simulink model "HESS"  (R2023a)
settings: Solver=daessc  StartTime=0.0  StopTime=1800  MaxStep=0.1  RelTol=1e-3
values from neighbouring files (symbols this model uses):
  Max_Power = 100000    [setHESSParam.m]    (also in setHESSParamv2.m)
  sim_case = i    [create_SOC_dataset.m]    (also in create_csv.m = 2; setHESSParam.m = 6; setHESSParamv2.m = 6)
undefined symbols (not defined in the file or in its folder): Battery, Capacitor, Ri
libraries: fl_lib x41, nesl_utility x22, rllib x2, dspstat3 x2, batteryecm_lib x1, autolibshared x1
(part 1 of 2)
settings Model: Creator=antaeug  LastModifiedBy=antaeug

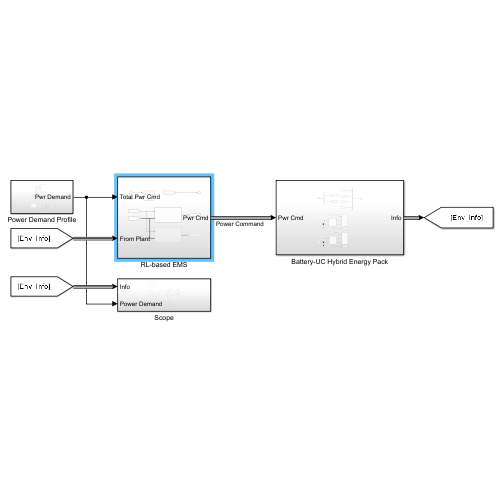
[thumbnail: Simulink's stored preview of the top-level diagram]
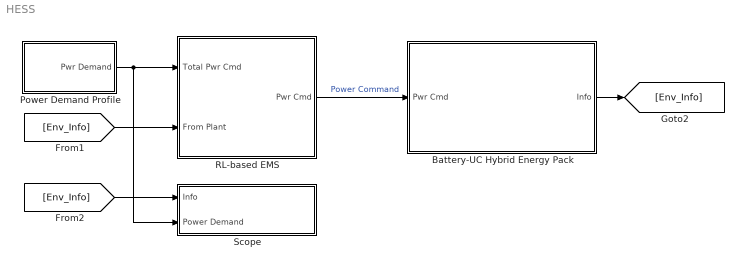
== system HESS ==
  Battery-UC Hybrid Energy Pack : Subsystem
  Power Demand Profile : Subsystem
  RL-based EMS : Subsystem
  Scope : Subsystem
  wires:
  Power Demand Profile/1(Pwr Demand) -> RL-based EMS/1(Total Pwr Cmd), Scope/2(Power Demand)
  RL-based EMS/1(Pwr Cmd) -> Battery-UC Hybrid Energy Pack/1(Pwr Cmd)  "Power Command"
  Battery-UC Hybrid Energy Pack/1(Info) -> [Env_Info]
  [Env_Info] -> Scope/1(Info)
  [Env_Info] -> RL-based EMS/2(From Plant)

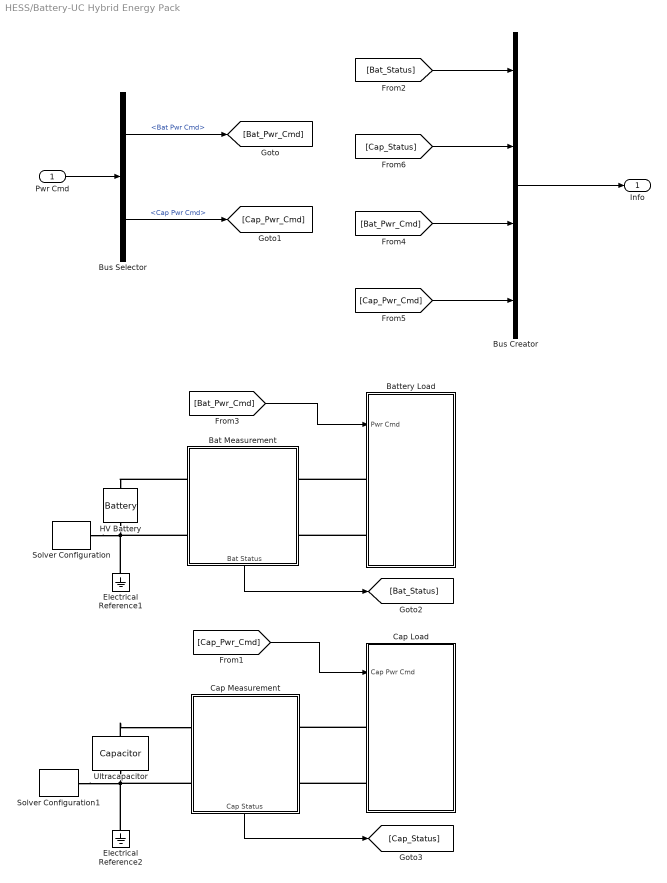
== system HESS/Battery-UC Hybrid Energy Pack ==
  Pwr Cmd : Inport
  Bat Measurement : Subsystem
      settings: PortSchema="{\"entries\":[{\"content\":{\"sides\":[{\"content\":{\"connectorIds\":[\"LConn1\",\"LConn2\"]},\"type\":\"ConnectorPlacement.EquallySpacedRectSide\",\"uuid\":\"d922d1f1-019d-451f-8be4-16b01e818775\"},{\"content\":{\"connectorIds\":[\"RConn1\",\"RConn2\"],\"side\":\"RIGHT\"},\"type\":\"ConnectorPlacement.EquallySpacedRectSide\",\"uuid\":\"6462d40f-4676-4bff-8e25-5b847feb4e24\"},{\"content\":{\"side\":\"TOP\"},\"type\":\"ConnectorPlacement.EquallySpacedRectSide\",\"uuid\":\"03ad4d94-013a-4b50-b094-3d1359848380\"},{\"content\":{\"connectorIds\":[\"Out1\"],\"side\":\"BOTTOM\"},\"type\":\"ConnectorPlacement.EquallySpacedRectSide\",\"uuid\":\"1e4082bc-bf86-4ee6-a4f5-78f09401198d\"}]},\"type\":\"ConnectorPlacement.EquallySpacedConnector\",\"uuid\":\"2964760f-0df3-43f8-9aa6-d9b794f3ad37\"}],\"packageUris\":[\"http://schema.mathworks.com/mf0/Connector/R2020b\"],\"version\":\"1.0\"}"
  Battery Load : Subsystem
  Bus Creator : BusCreator  Inputs=4
  Bus Selector : BusSelector  OutputSignals=Bat Pwr Cmd,Cap Pwr Cmd
  Cap Load : Subsystem
  Cap Measurement : Subsystem
      settings: PortSchema="{\"entries\":[{\"content\":{\"sides\":[{\"content\":{\"connectorIds\":[\"LConn1\",\"LConn2\"]},\"type\":\"ConnectorPlacement.EquallySpacedRectSide\",\"uuid\":\"d922d1f1-019d-451f-8be4-16b01e818775\"},{\"content\":{\"connectorIds\":[\"RConn1\",\"RConn2\"],\"side\":\"RIGHT\"},\"type\":\"ConnectorPlacement.EquallySpacedRectSide\",\"uuid\":\"6462d40f-4676-4bff-8e25-5b847feb4e24\"},{\"content\":{\"side\":\"TOP\"},\"type\":\"ConnectorPlacement.EquallySpacedRectSide\",\"uuid\":\"03ad4d94-013a-4b50-b094-3d1359848380\"},{\"content\":{\"connectorIds\":[\"Out1\"],\"side\":\"BOTTOM\"},\"type\":\"ConnectorPlacement.EquallySpacedRectSide\",\"uuid\":\"1e4082bc-bf86-4ee6-a4f5-78f09401198d\"}]},\"type\":\"ConnectorPlacement.EquallySpacedConnector\",\"uuid\":\"2964760f-0df3-43f8-9aa6-d9b794f3ad37\"}],\"packageUris\":[\"http://schema.mathworks.com/mf0/Connector/R2020b\"],\"version\":\"1.0\"}"
  Electrical Reference1 : fl_lib/Electrical/Electrical Elements/Electrical Reference
  Electrical Reference2 : fl_lib/Electrical/Electrical Elements/Electrical Reference
  HV Battery : batteryecm_lib/Battery  Vnom=Battery.NominalVoltage V  prm_dir=1  R1_dis=2 Ohm  R1_ch=2 Ohm  R1=Battery.InternalResistance Ohm  prm_AH=2  AH=Battery.Capacity hr*A  V1=Battery.V1 V  AH1=Battery.AH1 hr*A  prm_R2=simscape.enum.battery.prm_R2.disabled  R2=2000 Ohm  Tmeas=25 degC  charge_measurement_port=simscape.enum.battery.enable.no  prm_dyn=simscape.enum.battery.prm_dyn.off  Rp1=0.005 Ohm  tau1=30 s  Rp2=0.005 Ohm  tau2=30 s  Rp3=0.005 Ohm  tau3=30 s  Rp4=0.005 Ohm  tau4=30 s  Rp5=0.005 Ohm  tau5=30 s  prm_fade=simscape.enum.battery.prm_fade.disabled  N_fade=100  AH_fade=45 hr*A  R1_fade=2.02 Ohm  R1_ch_fade=2.02 Ohm  V1_fade=10.35 V  prm_age=simscape.enum.battery.prm_age.disabled  prm_age_OCV=1  OCV_age=0.9  SOC_age=60  Tmeas_age=298.15 K  delta_time_age_vec=[0] d  temperature_age_vec=[273] K  OCV_scaling_age=2.2134e6  OCV_offset_age=1.632e6  temp_exp_age=0.515833569 V  t_exp_age=0.75  Vnom_T2=Vnom V  R1_T2=Ri+0.1*Ri Ohm  R1_T2_dis=2.2 Ohm  R1_T2_ch=2.2 Ohm  V1_T2=V1 V  R2_T2=2200 Ohm  Rp1_T2=0.005 Ohm  tau1_T2=30 s  Rp2_T2=0.005 Ohm  tau2_T2=30 s  Rp3_T2=0.005 Ohm  tau3_T2=30 s  Rp4_T2=0.005 Ohm  tau4_T2=30 s  Rp5_T2=0.005 Ohm  tau5_T2=30 s  Tmeas2=0 degC  thermal_port=simscape.enum.thermaleffects.omit  thermal_mass=89400 J/K  i_specify=off  i_priority=None  i=0 A  i_nominal_specify=off  i_nominal_unit=A  i_nominal_value=1  v_specify=off  v_priority=None  v=0 V  v_nominal_specify=off  v_nominal_unit=V  v_nominal_value=1  charge_specify=on  charge_priority=High  charge=Battery.InitialCharge hr*A  charge_nominal_specify=off  charge_nominal_unit=A*hr  charge_nominal_value=1  num_cycles_specify=off  num_cycles_priority=High  num_cycles=0  num_cycles_nominal_specify=off  num_cycles_nominal_unit=1  num_cycles_nominal_value=1  temperature_specify=on  temperature_priority=High  temperature=25 degC  temperature_nominal_specify=off  temperature_nominal_unit=K  temperature_nominal_value=1
  Solver Configuration : nesl_utility/Solver Configuration  PhysicalDomain=network_engine_domain  SubClassName=solver  LeftPortType=input  RightPortType=generic  Tones=[]  Harmonics=[]  SimulateNoise=off  Profile=off  UseLocalSampling=off  EnableSwitchedLinearOptims=on  FrequencyDomain=off  UseCCode=off  RelTol=0.001  AbsTol=1e-06  MinStep=1e-09  ToWorkspace=off  RevertToSquareIcSolve=off  NumHomotopyIterations=100  PhasorMode=off  PhasorModeNumHarmonics=1  ConsistencySolver=NEWTON_FTOL  IndexReductionMethod=DerivativeReplacement  DoDC=off  ResidualTolerance=1e-09  ConsistencyTolSource=GLOBAL  ConsistencyAbsTol=0.001  ConsistencyRelTol=0.001  ConsistencyTolFactor=0.001  UseLocalSolver=on  LocalSolverChoice=NE_BACKWARD_EULER_ADVANCER  ResolveIndetEquations=on  FunctionEvalNumThread=1  LocalSolverSampleTime=0.01  DoFixedCost=on  MaxNonlinIter=3  MaxModeIter=2  ComputeImpulses=off  ImpulseIterations=2  LinearAlgebra=auto  LinearAlgebraNumThread=0  EquationFormulation=NE_TIME_EF  DelaysMemoryBudget=1024  AutomaticFiltering=on  FilteringTimeConstant=0.001  PartitionStorageMethod=AS_NEEDED  PartitionMemoryBudget=1024  PartitionMethod=FAST
  Solver Configuration1 : nesl_utility/Solver Configuration  PhysicalDomain=network_engine_domain  SubClassName=solver  LeftPortType=input  RightPortType=generic  Tones=[]  Harmonics=[]  SimulateNoise=off  Profile=off  UseLocalSampling=off  EnableSwitchedLinearOptims=on  FrequencyDomain=off  UseCCode=off  RelTol=0.001  AbsTol=1e-06  MinStep=1e-09  ToWorkspace=off  RevertToSquareIcSolve=off  NumHomotopyIterations=100  PhasorMode=off  PhasorModeNumHarmonics=1  ConsistencySolver=NEWTON_FTOL  IndexReductionMethod=DerivativeReplacement  DoDC=off  ResidualTolerance=1e-09  ConsistencyTolSource=GLOBAL  ConsistencyAbsTol=0.001  ConsistencyRelTol=0.001  ConsistencyTolFactor=0.001  UseLocalSolver=on  LocalSolverChoice=NE_BACKWARD_EULER_ADVANCER  ResolveIndetEquations=on  FunctionEvalNumThread=1  LocalSolverSampleTime=0.01  DoFixedCost=on  MaxNonlinIter=3  MaxModeIter=2  ComputeImpulses=off  ImpulseIterations=2  LinearAlgebra=auto  LinearAlgebraNumThread=0  EquationFormulation=NE_TIME_EF  DelaysMemoryBudget=1024  AutomaticFiltering=on  FilteringTimeConstant=0.001  PartitionStorageMethod=AS_NEEDED  PartitionMemoryBudget=1024  PartitionMethod=FAST
  Ultracapacitor : fl_lib/Electrical/Electrical Elements/Capacitor  c=Capacitor.Capacitance F  r=Capacitor.InternalResistance mOhm  g=0 1/Ohm  i_specify=off  i_priority=None  i=20 A  i_nominal_specify=off  i_nominal_unit=A  i_nominal_value=1  v_specify=off  v_priority=None  v=600 V  v_nominal_specify=off  v_nominal_unit=V  v_nominal_value=1  vc_specify=on  vc_priority=None  vc=Capacitor.Voltage V  vc_nominal_specify=off  vc_nominal_unit=V  vc_nominal_value=600
  Info : Outport
  wires:
  Pwr Cmd/1 -> Bus Selector/1
  Bus Selector/1 -> [Bat_Pwr_Cmd]  "<Bat Pwr Cmd>"
  Bus Selector/2 -> [Cap_Pwr_Cmd]  "<Cap Pwr Cmd>"
  [Bat_Status] -> Bus Creator/1
  Bus Creator/1 -> Info/1
  [Cap_Pwr_Cmd] -> Bus Creator/4
  [Bat_Pwr_Cmd] -> Bus Creator/3
  Bat Measurement/1(Bat Status) -> [Bat_Status]
  [Bat_Pwr_Cmd] -> Battery Load/1(Pwr Cmd)
  Cap Measurement/1(Cap Status) -> [Cap_Status]
  [Cap_Pwr_Cmd] -> Cap Load/1(Cap Pwr Cmd)
  [Cap_Status] -> Bus Creator/2
  connections:
  HV Battery/RConn1 -- Solver Configuration/RConn1 -- Electrical Reference1/LConn1 -- Bat Measurement/LConn2
  Bat Measurement/LConn1 -- HV Battery/LConn1
  Battery Load/LConn1 -- Bat Measurement/RConn1
  Battery Load/LConn2 -- Bat Measurement/RConn2
  Electrical Reference2/LConn1 -- Ultracapacitor/RConn1 -- Solver Configuration1/RConn1 -- Cap Measurement/LConn2
  Ultracapacitor/LConn1 -- Cap Measurement/LConn1
  Cap Load/LConn2 -- Cap Measurement/RConn2
  Cap Load/LConn1 -- Cap Measurement/RConn1

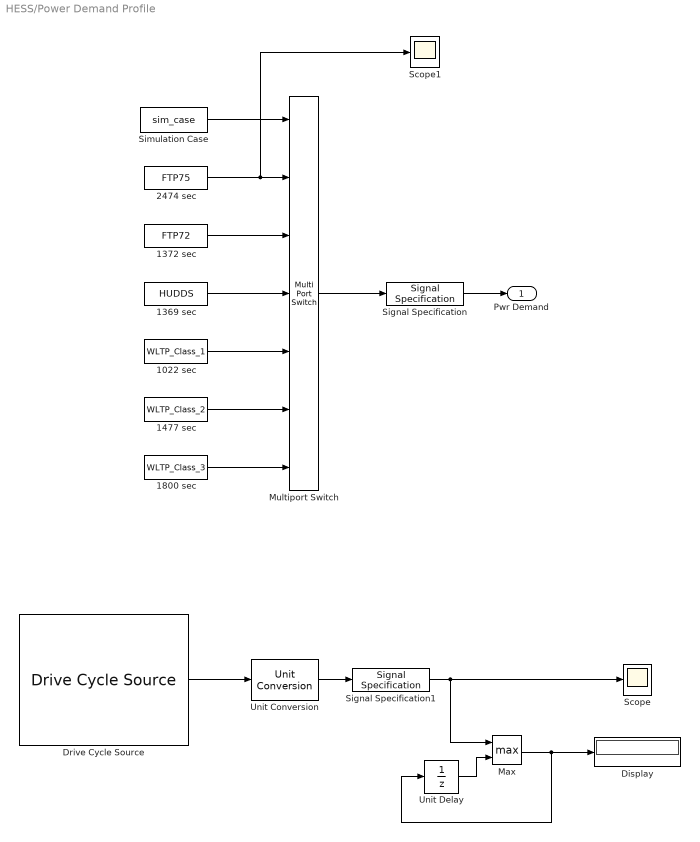
== system HESS/Power Demand Profile ==
  1022 sec : FromWorkspace  VariableName=WLTP_Class_1  Interpolate=off  ZeroCross=off  OutputAfterFinalValue=Setting to zero
  1369 sec : FromWorkspace  VariableName=HUDDS  Interpolate=off  ZeroCross=off  OutputAfterFinalValue=Setting to zero
  1372 sec : FromWorkspace  VariableName=FTP72  Interpolate=off  ZeroCross=off  OutputAfterFinalValue=Setting to zero
  1477 sec : FromWorkspace  VariableName=WLTP_Class_2  Interpolate=off  ZeroCross=off  OutputAfterFinalValue=Setting to zero
  1800 sec : FromWorkspace  VariableName=WLTP_Class_3  Interpolate=off  ZeroCross=off  OutputAfterFinalValue=Setting to zero
  2474 sec : FromWorkspace  VariableName=FTP75  Interpolate=off  ZeroCross=off  OutputAfterFinalValue=Setting to zero
  Display : Display
  Drive Cycle Source : autolibshared/Drive Cycle Source  cycleVar=Artemis Rural Road  fileVar=cycleFTP75.mat  tfinal="1082  seconds"  cycleRepeat=off  outAccPort=off  outGearPort=off  gearList=No gear data  t_wot1=5  xdot_woto=0  xdot_wot1=30  t_wot2=20  xdot_wot2=0  t_wotend=30  srcUnit=m/s  outUnit=m/s  srcAccUnit=m/s/s  outAccUnit=m/s^2  dt=0  aMode=1  faultOption=off  velBnd=2  velBndUnit=mph  inUnit=m/s  timeBnd=1  failOption=off  stopSim=off  maxFaultCnt=10  maxFaultTime=2  maxTotFaultTime=15  traceOption=off  dtTrace=1  traceWindow=10  lastDCname=Artemis Rural Road  lastOutUnit=mph  lastDT=0  lastTB=1  lastSB=2  forceCalcBound=off
  Max : MinMax  Function=max  Inputs=2
  Multiport Switch : MultiPortSwitch  Inputs=6  SaturateOnIntegerOverflow=off  InputSameDT=off
  Scope : Scope
  Scope1 : Scope
  Signal Specification : SignalSpecification  Unit=W
  Signal Specification1 : SignalSpecification  Unit=km/h
  Simulation Case : Constant  Value=sim_case
  Unit Conversion : UnitConversion
  Unit Delay : UnitDelay  SampleTime=-1  HasFrameUpgradeWarning=on
  Pwr Demand : Outport
  wires:
  2474 sec/1 -> Scope1/1, Multiport Switch/2
  Signal Specification/1 -> Pwr Demand/1
  Multiport Switch/1 -> Signal Specification/1
  Simulation Case/1 -> Multiport Switch/1
  1372 sec/1 -> Multiport Switch/3
  1369 sec/1 -> Multiport Switch/4
  1477 sec/1 -> Multiport Switch/6
  1022 sec/1 -> Multiport Switch/5
  1800 sec/1 -> Multiport Switch/7
  Drive Cycle Source/1 -> Unit Conversion/1
  Unit Conversion/1 -> Signal Specification1/1
  Signal Specification1/1 -> Max/1, Scope/1
  Max/1 -> Display/1, Unit Delay/1
  Unit Delay/1 -> Max/2

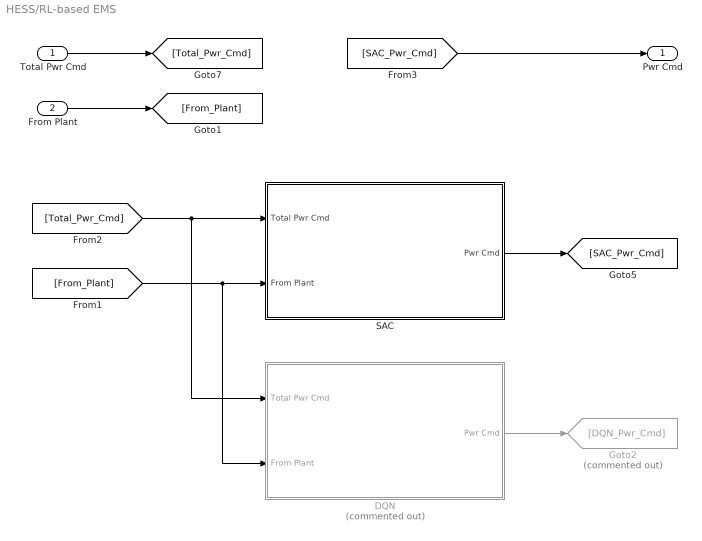
== system HESS/RL-based EMS ==
  Total Pwr Cmd : Inport
  From Plant : Inport  Port=2
  DQN : Subsystem  Commented=on
  Goto2 : Goto  Commented=on  GotoTag=DQN_Pwr_Cmd
  SAC : Subsystem
  Pwr Cmd : Outport
  wires:
  [Total_Pwr_Cmd] -> SAC/1(Total Pwr Cmd), DQN/1(Total Pwr Cmd)
  Total Pwr Cmd/1 -> [Total_Pwr_Cmd]
  From Plant/1 -> [From_Plant]
  [SAC_Pwr_Cmd] -> Pwr Cmd/1
  [From_Plant] -> DQN/2(From Plant), SAC/2(From Plant)
  SAC/1(Pwr Cmd) -> [SAC_Pwr_Cmd]
  DQN/1(Pwr Cmd) -> Goto2/1

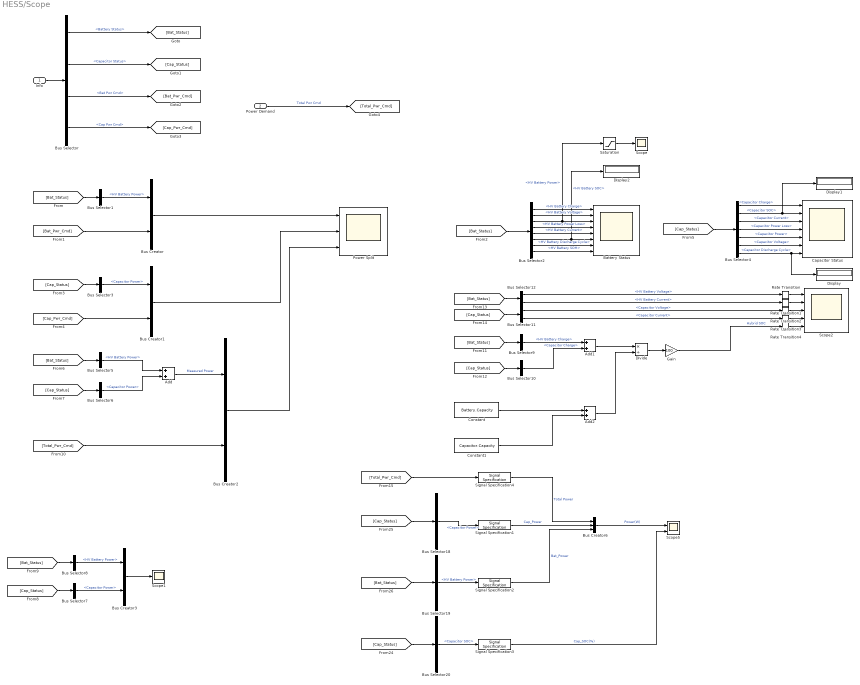
== system HESS/Scope ==
  Info : Inport
  Power Demand : Inport  Port=2
  Add : Sum
  Add1 : Sum
  Add2 : Sum
  Battery Status : Scope  NumInputPorts=8
  Bus Creator{,1..3} (4 alike) : BusCreator  Inputs=2
  Bus Creator6 : BusCreator  Inputs=3
  Bus Selector : BusSelector  OutputSignals=Battery Status,Capacitor Status,Bat Pwr Cmd,Cap Pwr Cmd
  Bus Selector{1,5,8,19} (4 alike) : BusSelector  OutputSignals=HV Battery Power
  Bus Selector10 : BusSelector  OutputSignals=Capacitor Charge
  Bus Selector11 : BusSelector  OutputSignals=Capacitor Voltage,Capacitor Current
  Bus Selector12 : BusSelector  OutputSignals=HV Battery Voltage,HV Battery Current
  Bus Selector{3,6..7,18} (4 alike) : BusSelector  OutputSignals=Capacitor Power
  Bus Selector2 : BusSelector  OutputSignals=HV Battery Charge,HV Battery Voltage,HV Battery Power,HV Battery Power Loss,HV Battery Current,HV Battery SOC,HV Battery Discharge Cycle,HV Battery SOH
  Bus Selector20 : BusSelector  OutputSignals=Capacitor SOC
  Bus Selector4 : BusSelector  OutputSignals=Capacitor Charge,Capacitor SOC,Capacitor Current,Capacitor Power Loss,Capacitor Power,Capacitor Voltage,Capacitor Discharge Cycle
  Bus Selector9 : BusSelector  OutputSignals=HV Battery Charge
  Capacitor Status : Scope  NumInputPorts=7
  Constant : Constant  Value=Battery.Capacity
  Constant1 : Constant  Value=Capacitor.Capacity
  Display : Display
  Display1 : Display
  Display2 : Display
  Divide : Product  Inputs=*/
  Gain : Gain  Gain=100
  Power Split : Scope  NumInputPorts=3
  Rate Transition{,1..4} (5 alike) : RateTransition  OutPortSampleTime=0.5
  Saturation : Saturate  UpperLimit=200000  LowerLimit=0
  Scope : Scope
  Scope1 : Scope
  Scope2 : Scope  NumInputPorts=5
  Scope5 : Scope  NumInputPorts=2
  Signal Specification1 : SignalSpecification  Unit=W
  Signal Specification2 : SignalSpecification  Unit=W
  Signal Specification3 : SignalSpecification  Unit=%
  Signal Specification4 : SignalSpecification  Unit=W
  wires:
  Info/1 -> Bus Selector/1
  Bus Selector/1 -> [Bat_Status]  "<Battery Status>"
  [Bat_Status] -> Bus Selector1/1
  Bus Selector1/1 -> Bus Creator/1  "<HV Battery Power>"
  [Bat_Pwr_Cmd] -> Bus Creator/2
  Bus Selector/3 -> [Bat_Pwr_Cmd]  "<Bat Pwr Cmd>"
  Bus Selector/4 -> [Cap_Pwr_Cmd]  "<Cap Pwr Cmd>"
  [Bat_Status] -> Bus Selector2/1
  Bus Selector2/1 -> Battery Status/1  "<HV Battery Charge>"
  Bus Selector2/2 -> Battery Status/2  "<HV Battery Voltage>"
  Bus Selector2/3 -> Saturation/1, Battery Status/3  "<HV Battery Power>"
  Bus Selector2/4 -> Battery Status/4  "<HV Battery Power Loss>"
  Bus Selector2/5 -> Battery Status/5  "<HV Battery Current>"
  Bus Selector2/6 -> Display2/1, Battery Status/6  "<HV Battery SOC>"
  Bus Selector3/1 -> Bus Creator1/1  "<Capacitor Power>"
  [Cap_Status] -> Bus Selector3/1
  [Cap_Pwr_Cmd] -> Bus Creator1/2
  Bus Selector/2 -> [Cap_Status]  "<Capacitor Status>"
  Bus Creator/1 -> Power Split/1
  Bus Creator1/1 -> Power Split/2
  Bus Selector4/6 -> Capacitor Status/6  "<Capacitor Voltage>"
  Bus Selector4/1 -> Capacitor Status/1  "<Capacitor Charge>"
  Bus Selector4/2 -> Display1/1, Capacitor Status/2  "<Capacitor SOC>"
  Bus Selector4/3 -> Capacitor Status/3  "<Capacitor Current>"
  Bus Selector4/4 -> Capacitor Status/4  "<Capacitor Power Loss>"
  Bus Selector4/5 -> Capacitor Status/5  "<Capacitor Power>"
  [Cap_Status] -> Bus Selector4/1
  [Bat_Status] -> Bus Selector5/1
  [Cap_Status] -> Bus Selector6/1
  Bus Selector5/1 -> Add/1  "<HV Battery Power>"
  Add/1 -> Bus Creator2/1  "Measured Power"
  Bus Selector6/1 -> Add/2  "<Capacitor Power>"
  Bus Creator2/1 -> Power Split/3
  Power Demand/1 -> [Total_Pwr_Cmd]  "Total Pwr Cmd"
  [Total_Pwr_Cmd] -> Bus Creator2/2
  Bus Selector2/7 -> Battery Status/7  "<HV Battery Discharge Cycle>"
  Bus Selector2/8 -> Battery Status/8  "<HV Battery SOH>"
  Bus Selector4/7 -> Display/1, Capacitor Status/7  "<Capacitor Discharge Cycle>"
  [Cap_Status] -> Bus Selector7/1
  Bus Selector7/1 -> Bus Creator3/2  "<Capacitor Power>"
  Bus Selector8/1 -> Bus Creator3/1  "<HV Battery Power>"
  [Bat_Status] -> Bus Selector8/1
  Bus Creator3/1 -> Scope1/1
  [Bat_Status] -> Bus Selector9/1
  Bus Selector9/1 -> Add1/1  "<HV Battery Charge>"
  Bus Selector10/1 -> Add1/2  "<Capacitor Charge>"
  [Cap_Status] -> Bus Selector10/1
  Constant/1 -> Add2/1
  Constant1/1 -> Add2/2
  Add1/1 -> Divide/1
  Add2/1 -> Divide/2
  Divide/1 -> Gain/1
  Gain/1 -> Rate Transition4/1  "Hybrid SOC"
  [Cap_Status] -> Bus Selector11/1
  [Bat_Status] -> Bus Selector12/1
  Bus Selector12/1 -> Rate Transition/1  "<HV Battery Voltage>"
  Bus Selector12/2 -> Rate Transition1/1  "<HV Battery Current>"
  Bus Selector11/1 -> Rate Transition2/1  "<Capacitor Voltage>"
  Bus Selector11/2 -> Rate Transition3/1  "<Capacitor Current>"
  [Cap_Status] -> Bus Selector18/1
  [Bat_Status] -> Bus Selector19/1
  Bus Selector19/1 -> Signal Specification2/1  "<HV Battery Power>"
  Bus Selector18/1 -> Signal Specification1/1  "<Capacitor Power>"
  Bus Creator6/1 -> Scope5/1  "Power(W)"
  [Cap_Status] -> Bus Selector20/1
  Bus Selector20/1 -> Signal Specification3/1  "<Capacitor SOC>"
  Signal Specification3/1 -> Scope5/2  "Cap_SOC(%)"
  Rate Transition/1 -> Scope2/1
  Rate Transition1/1 -> Scope2/2
  Rate Transition2/1 -> Scope2/3
  Rate Transition3/1 -> Scope2/4
  Rate Transition4/1 -> Scope2/5
  Signal Specification1/1 -> Bus Creator6/2  "Cap_Power"
  Signal Specification2/1 -> Bus Creator6/3  "Bat_Power"
  [Total_Pwr_Cmd] -> Signal Specification4/1
  Signal Specification4/1 -> Bus Creator6/1  "Total Power"
  Saturation/1 -> Scope/1

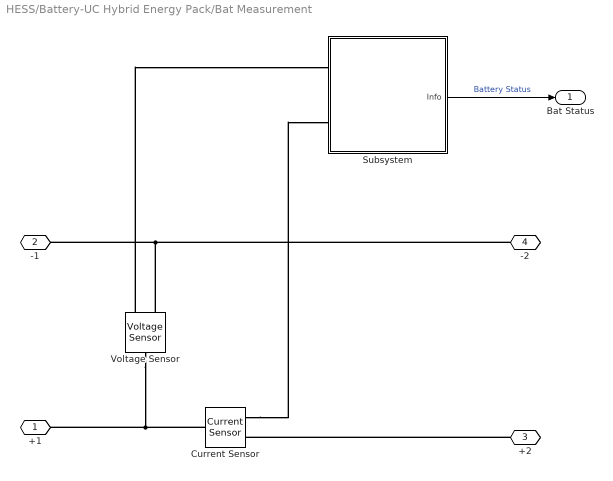
== system HESS/Battery-UC Hybrid Energy Pack/Bat Measurement ==
  Current Sensor : fl_lib/Electrical/Electrical Sensors/Current Sensor
  Subsystem : Subsystem
  Voltage Sensor : fl_lib/Electrical/Electrical Sensors/Voltage Sensor
  +1 : PMIOPort  Side=Left
  -1 : PMIOPort  Port=2  Side=Left
  +2 : PMIOPort  Port=3  Side=Right
  -2 : PMIOPort  Port=4  Side=Right
  Bat Status : Outport
  wires:
  Subsystem/1(Info) -> Bat Status/1  "Battery Status"
  connections:
  Voltage Sensor/RConn2 -- -1/RConn1 -- -2/RConn1
  Current Sensor/LConn1 -- Voltage Sensor/LConn1 -- +1/RConn1
  Voltage Sensor/RConn1 -- Subsystem/LConn1
  Current Sensor/RConn1 -- Subsystem/LConn2
  +2/RConn1 -- Current Sensor/RConn2

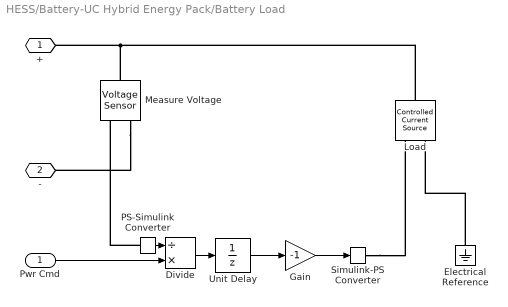
== system HESS/Battery-UC Hybrid Energy Pack/Battery Load ==
  Pwr Cmd : Inport
  Divide : Product  Inputs=/*
  Electrical Reference : fl_lib/Electrical/Electrical Elements/Electrical Reference
  Gain : Gain  Gain=-1
  Load : fl_lib/Electrical/Electrical Sources/Controlled Current Source
  Measure Voltage : fl_lib/Electrical/Electrical Sensors/Voltage Sensor
  PS-Simulink Converter : nesl_utility/PS-Simulink Converter  PhysicalDomain=network_engine_domain  SubClassName=ps_output  LeftPortType=input  RightPortType=output  PseudoPeriodic=off  Frequencies=[]  VectorFormat=inherit  Unit=V  AffineConversion=off
  Simulink-PS Converter : nesl_utility/Simulink-PS Converter  PhysicalDomain=network_engine_domain  SubClassName=ps_input  LeftPortType=input  RightPortType=output  PseudoPeriodic=off  Frequencies=[]  NoiseDistribution=none  NoiseParameters=[]  Unit=A  AffineConversion=off  FilteringAndDerivatives=provide  SimscapeFilterOrder=1  InputFilterTimeConstant=0.001  UdotUserProvided=0
  Unit Delay : UnitDelay  SampleTime=-1  HasFrameUpgradeWarning=on
  + : PMIOPort  Side=Left
  - : PMIOPort  Port=2  Side=Left
  wires:
  PS-Simulink Converter/1 -> Divide/1
  Pwr Cmd/1 -> Divide/2
  Divide/1 -> Unit Delay/1
  Unit Delay/1 -> Gain/1
  Gain/1 -> Simulink-PS Converter/1
  connections:
  Electrical Reference/LConn1 -- Load/RConn2
  Load/LConn1 -- Measure Voltage/LConn1 -- +/RConn1
  Measure Voltage/RConn2 -- -/RConn1
  PS-Simulink Converter/LConn1 -- Measure Voltage/RConn1
  Simulink-PS Converter/RConn1 -- Load/RConn1

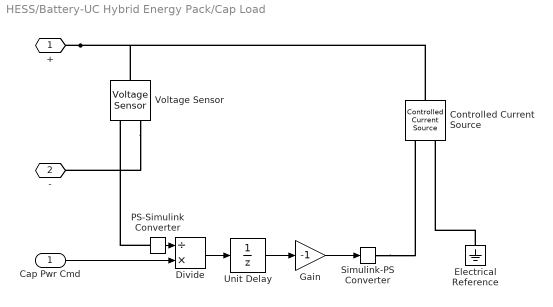
== system HESS/Battery-UC Hybrid Energy Pack/Cap Load ==
  Cap Pwr Cmd : Inport
  Controlled Current Source : fl_lib/Electrical/Electrical Sources/Controlled Current Source
  Divide : Product  Inputs=/*
  Electrical Reference : fl_lib/Electrical/Electrical Elements/Electrical Reference
  Gain : Gain  Gain=-1
  PS-Simulink Converter : nesl_utility/PS-Simulink Converter  PhysicalDomain=network_engine_domain  SubClassName=ps_output  LeftPortType=input  RightPortType=output  PseudoPeriodic=off  Frequencies=[]  VectorFormat=inherit  Unit=V  AffineConversion=off
  Simulink-PS Converter : nesl_utility/Simulink-PS Converter  PhysicalDomain=network_engine_domain  SubClassName=ps_input  LeftPortType=input  RightPortType=output  PseudoPeriodic=off  Frequencies=[]  NoiseDistribution=none  NoiseParameters=[]  Unit=A  AffineConversion=off  FilteringAndDerivatives=provide  SimscapeFilterOrder=1  InputFilterTimeConstant=0.001  UdotUserProvided=0
  Unit Delay : UnitDelay  SampleTime=-1  HasFrameUpgradeWarning=on
  Voltage Sensor : fl_lib/Electrical/Electrical Sensors/Voltage Sensor
  + : PMIOPort  Side=Left
  - : PMIOPort  Port=2  Side=Left
  wires:
  PS-Simulink Converter/1 -> Divide/1
  Cap Pwr Cmd/1 -> Divide/2
  Divide/1 -> Unit Delay/1
  Unit Delay/1 -> Gain/1
  Gain/1 -> Simulink-PS Converter/1
  connections:
  Electrical Reference/LConn1 -- Controlled Current Source/RConn2
  +/RConn1 -- Controlled Current Source/LConn1 -- Voltage Sensor/LConn1
  Voltage Sensor/RConn2 -- -/RConn1
  PS-Simulink Converter/LConn1 -- Voltage Sensor/RConn1
  Simulink-PS Converter/RConn1 -- Controlled Current Source/RConn1

== system HESS/Battery-UC Hybrid Energy Pack/Cap Measurement ==
  Current Sensor : fl_lib/Electrical/Electrical Sensors/Current Sensor
  Subsystem : Subsystem
  Voltage Sensor : fl_lib/Electrical/Electrical Sensors/Voltage Sensor
  +1 : PMIOPort  Side=Left
  -1 : PMIOPort  Port=2  Side=Left
  +2 : PMIOPort  Port=3  Side=Right
  -2 : PMIOPort  Port=4  Side=Right
  Cap Status : Outport
  wires:
  Subsystem/1(Info) -> Cap Status/1  "Capacitor Status"
  connections:
  -2/RConn1 -- Voltage Sensor/RConn2 -- -1/RConn1
  Current Sensor/LConn1 -- Voltage Sensor/LConn1 -- +1/RConn1
  Voltage Sensor/RConn1 -- Subsystem/LConn1
  Current Sensor/RConn1 -- Subsystem/LConn2
  +2/RConn1 -- Current Sensor/RConn2

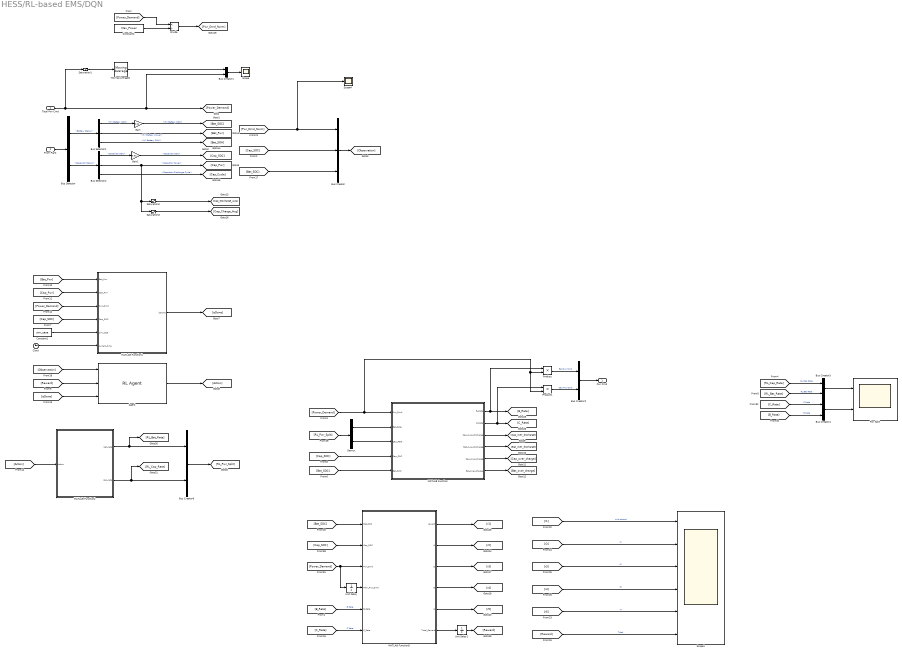
== system HESS/RL-based EMS/DQN ==
  Total Pwr Cmd : Inport
  From Plant : Inport  Port=2
  Agent : rllib/RL Agent  Agent=saved_agent  ExternalActionAsInput=off  ProvideLastAction=off  ProvideCumRwd=off  TreatAsDirectFeedthrough=on  UseStrictObservationDataTypes=off
  Bus Creator : BusCreator  Inputs=3
  Bus Creator{1..4,6} (5 alike) : BusCreator  Inputs=2
  Bus Selector : BusSelector  OutputSignals=Battery Status,Capacitor Status
  Bus Selector1 : BusSelector  OutputSignals=HV Battery SOC,HV Battery Power,HV Battery SOH
  Bus Selector2 : BusSelector  OutputSignals=Capacitor SOC,Capacitor Power,Capacitor Discharge Cycle
  Clock : Clock
  Constant1 : Constant  Value=sim_case
  Constant2 : Constant  Value=Max_Power
  Demux : Demux  Outputs=2
  Divide : Product  Inputs=*/
  Gain : Gain  Gain=0.01
  Gain1 : Gain  Gain=0.01
  MATLAB Function : MATLAB Function  TreatAsAtomicUnit=on
  MATLAB Function1 : MATLAB Function  TreatAsAtomicUnit=on
  MATLAB Function2 : MATLAB Function  TreatAsAtomicUnit=on
  MATLAB Function5 : MATLAB Function  TreatAsAtomicUnit=on
  Moving Average1 : dspstat3/Moving Average  Method=Exponential weighting  ForgettingFactorPort=off  SpecifyWindowLength=on  WindowLength=4  OverlapLength=3  AllowArbitraryInputLength=off  ForgettingFactor=0.9995  SimulateUsing=Code generation
  Product : Product
  Product1 : Product
  Pwr Split : Scope  NumInputPorts=2
  Saturation1 : Saturate  UpperLimit=200000  LowerLimit=0
  Saturation2 : Saturate  UpperLimit=200000  LowerLimit=0
  Saturation3 : Saturate  UpperLimit=0  LowerLimit=-200000
  Scope : Scope
  Scope1 : Scope  NumInputPorts=6
  Scope4 : Scope
  Unit Delay : UnitDelay  SampleTime=-1  HasFrameUpgradeWarning=on
  Unit Delay1 : UnitDelay  SampleTime=-1  HasFrameUpgradeWarning=on
  Pwr Cmd : Outport
  wires:
  From Plant/1 -> Bus Selector/1
  Total Pwr Cmd/1 -> Saturation1/1, Bus Creator1/2, [Power_Demand]
  Bus Selector/1 -> Bus Selector1/1  "<Battery Status>"
  Bus Selector/2 -> Bus Selector2/1  "<Capacitor Status>"
  Bus Selector1/1 -> Gain/1  "<HV Battery SOC>"
  Bus Creator/1 -> [Observation]
  Bus Selector1/2 -> [Bat_Pwr]  "<HV Battery Power>"
  Bus Selector2/1 -> Gain1/1  "<Capacitor SOC>"
  Bus Selector2/2 -> [Cap_Pwr], Saturation3/1, Saturation2/1  "<Capacitor Power>"
  [Bat_Pwr] -> MATLAB Function1/1(Bat_Pwr)
  [Cap_Pwr] -> MATLAB Function1/2(Cap_Pwr)
  [Power_Demand] -> MATLAB Function1/3(Pwr_Dmd)
  MATLAB Function1/1(isDone) -> [isDone]
  Bus Creator2/1 -> Pwr Cmd/1
  Gain/1 -> [Bat_SOC]  "<HV Battery SOC>"
  Gain1/1 -> [Cap_SOC]  "<Capacitor SOC>"
  [Cap_SOC] -> MATLAB Function1/4(Cap_SOC)
  Bus Selector1/3 -> [Bat_SOH]  "<HV Battery SOH>"
  Bus Selector2/3 -> [Cap_Cycle]  "<Capacitor Discharge Cycle>"
  [Cap_SOC] -> Bus Creator/2
  [Cap_SOC] -> MATLAB Function5/2(Cap_SOC)
  MATLAB Function5/1(reward) -> [r1]
  [Power_Demand] -> Unit Delay/1, MATLAB Function5/3(Pwr_Dmd)
  MATLAB Function5/2(r1) -> [r2]
  Product/1 -> Bus Creator2/1  "Bat Pwr Cmd"
  Product1/1 -> Bus Creator2/2  "Cap Pwr Cmd"
  Agent/1 -> [Action]
  [RL_Cap_Rate] -> Bus Creator3/1  "RL Cap Rate"
  [RL_Bat_Rate] -> Bus Creator3/2  "RL Bat Rate"
  Bus Creator3/1 -> Pwr Split/1
  Bus Creator6/1 -> [RL_Pwr_Split]
  [Power_Demand] -> MATLAB Function/1(Pwr_Dmd), Product1/2, Product/2
  Saturation2/1 -> [Cap_Discharge_Avg]
  [RL_Pwr_Split] -> Demux/1
  Demux/1 -> MATLAB Function/2(Bat_Rate)
  Demux/2 -> MATLAB Function/3(Cap_Rate)
  [Cap_SOC] -> MATLAB Function/4(Cap_SOC)
  [Bat_SOC] -> MATLAB Function/5(Bat_SOC)
  MATLAB Function/1(B_Rate) -> [B_Rate], Product/1
  MATLAB Function/2(C_Rate) -> [C_Rate], Product1/1
  MATLAB Function/3(Cap_over_discharge) -> [Cap_over_discharge]
  MATLAB Function/4(Bat_over_discharge) -> [Bat_over_discharge]
  MATLAB Function/5(Cap_over_charge) -> [Cap_over_charge]
  MATLAB Function/6(Bat_over_charge) -> [Bat_over_charge]
  Saturation3/1 -> [Cap_Charge_Avg]
  MATLAB Function5/3(r2) -> [r3]
  MATLAB Function5/4(r3) -> [r4]
  MATLAB Function5/6(Total_Reward) -> Unit Delay1/1
  [r1] -> Scope1/1  "mid reward"
  [r2] -> Scope1/2  "r1"
  [r3] -> Scope1/3  "r2"
  [r4] -> Scope1/4  "r3"
  [Reward] -> Scope1/6  "Total"
  Unit Delay1/1 -> [Reward]
  [C_Rate] -> Bus Creator4/1  "C Rate"
  [B_Rate] -> Bus Creator4/2  "B Rate"
  Bus Creator4/1 -> Pwr Split/2
  [Observation] -> Agent/1
  [Reward] -> Agent/2
  [isDone] -> Agent/3
  MATLAB Function2/2(cap_rate) -> [RL_Cap_Rate], Bus Creator6/2
  MATLAB Function2/1(bat_rate) -> [RL_Bat_Rate], Bus Creator6/1
  Constant1/1 -> MATLAB Function1/5(sim_case)
  Clock/1 -> MATLAB Function1/6(current_time)
  Constant2/1 -> Divide/2
  [B_Rate] -> MATLAB Function5/5(B_Rate)  "B Rate"
  [C_Rate] -> MATLAB Function5/6(C_Rate)  "C Rate"
  [Bat_SOC] -> Bus Creator/3
  [Power_Demand] -> Divide/1
  [Pwr_Dmd_Norm] -> Scope4/1, Bus Creator/1
  [Bat_SOC] -> MATLAB Function5/1(Bat_SOC)
  Moving Average1/1 -> Bus Creator1/1
  Bus Creator1/1 -> Scope/1
  Saturation1/1 -> Moving Average1/1
  Divide/1 -> [Pwr_Dmd_Norm]
  Unit Delay/1 -> MATLAB Function5/4(Prev_Pwr_Dmd)
  MATLAB Function5/5(r4) -> [r5]
  [r5] -> Scope1/5  "r4"
  [Action] -> MATLAB Function2/1(Action)

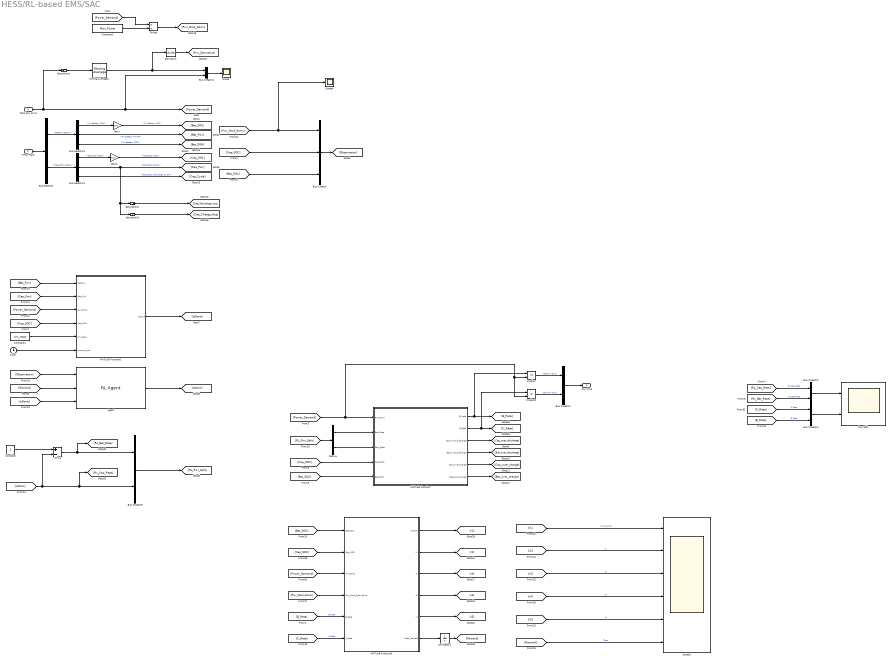
== system HESS/RL-based EMS/SAC ==
  Total Pwr Cmd : Inport
  From Plant : Inport  Port=2
  Agent : rllib/RL Agent  Agent=saved_agent  ExternalActionAsInput=off  ProvideLastAction=off  ProvideCumRwd=off  TreatAsDirectFeedthrough=on  UseStrictObservationDataTypes=off
  Bus Creator : BusCreator  Inputs=3
  Bus Creator{1..4,6} (5 alike) : BusCreator  Inputs=2
  Bus Selector : BusSelector  OutputSignals=Battery Status,Capacitor Status
  Bus Selector1 : BusSelector  OutputSignals=HV Battery SOC,HV Battery Power,HV Battery SOH
  Bus Selector2 : BusSelector  OutputSignals=Capacitor SOC,Capacitor Power,Capacitor Discharge Cycle
  Clock : Clock
  Constant : Constant
  Constant1 : Constant  Value=sim_case
  Constant2 : Constant  Value=Max_Power
  Demux : Demux  Outputs=2
  Derivative : Derivative
  Divide : Product  Inputs=*/
  Gain : Gain  Gain=0.01
  Gain1 : Gain  Gain=0.01
  MATLAB Function : MATLAB Function  TreatAsAtomicUnit=on
  MATLAB Function1 : MATLAB Function  TreatAsAtomicUnit=on
  MATLAB Function5 : MATLAB Function  TreatAsAtomicUnit=on
  Minus : Sum  Inputs=+-
  Moving Average1 : dspstat3/Moving Average  Method=Exponential weighting  ForgettingFactorPort=off  SpecifyWindowLength=on  WindowLength=4  OverlapLength=3  AllowArbitraryInputLength=off  ForgettingFactor=0.9995  SimulateUsing=Code generation
  Product : Product
  Product1 : Product
  Pwr Split : Scope  NumInputPorts=2
  Saturation1 : Saturate  UpperLimit=200000  LowerLimit=0
  Saturation2 : Saturate  UpperLimit=200000  LowerLimit=0
  Saturation3 : Saturate  UpperLimit=0  LowerLimit=-200000
  Scope : Scope
  Scope1 : Scope  NumInputPorts=6
  Scope4 : Scope
  Unit Delay1 : UnitDelay  SampleTime=-1  HasFrameUpgradeWarning=on
  Pwr Cmd : Outport
  wires:
  From Plant/1 -> Bus Selector/1
  Total Pwr Cmd/1 -> Saturation1/1, Bus Creator1/2, [Power_Demand]
  Bus Selector/1 -> Bus Selector1/1  "<Battery Status>"
  Bus Selector/2 -> Bus Selector2/1  "<Capacitor Status>"
  Bus Selector1/1 -> Gain/1  "<HV Battery SOC>"
  Bus Creator/1 -> [Observation]
  Bus Selector1/2 -> [Bat_Pwr]  "<HV Battery Power>"
  Bus Selector2/1 -> Gain1/1  "<Capacitor SOC>"
  Bus Selector2/2 -> [Cap_Pwr], Saturation3/1, Saturation2/1  "<Capacitor Power>"
  [Bat_Pwr] -> MATLAB Function1/1(Bat_Pwr)
  [Cap_Pwr] -> MATLAB Function1/2(Cap_Pwr)
  [Power_Demand] -> MATLAB Function1/3(Pwr_Dmd)
  MATLAB Function1/1(isDone) -> [isDone]
  Bus Creator2/1 -> Pwr Cmd/1
  Gain/1 -> [Bat_SOC]  "<HV Battery SOC>"
  Gain1/1 -> [Cap_SOC]  "<Capacitor SOC>"
  [Cap_SOC] -> MATLAB Function1/4(Cap_SOC)
  Bus Selector1/3 -> [Bat_SOH]  "<HV Battery SOH>"
  Bus Selector2/3 -> [Cap_Cycle]  "<Capacitor Discharge Cycle>"
  [Cap_SOC] -> Bus Creator/2
  [Cap_SOC] -> MATLAB Function5/2(Cap_SOC)
  MATLAB Function5/1(reward) -> [r1]
  [Power_Demand] -> MATLAB Function5/3(Pwr_Dmd)
  MATLAB Function5/2(r1) -> [r2]
  Product/1 -> Bus Creator2/1  "Bat Pwr Cmd"
  Product1/1 -> Bus Creator2/2  "Cap Pwr Cmd"
  Agent/1 -> [Action]
  Constant/1 -> Minus/1
  [RL_Cap_Rate] -> Bus Creator3/1  "RL Cap Rate"
  [RL_Bat_Rate] -> Bus Creator3/2  "RL Bat Rate"
  Bus Creator3/1 -> Pwr Split/1
  Bus Creator6/1 -> [RL_Pwr_Split]
  [Power_Demand] -> MATLAB Function/1(Pwr_Dmd), Product1/2, Product/2
  Saturation2/1 -> [Cap_Discharge_Avg]
  [RL_Pwr_Split] -> Demux/1
  Demux/1 -> MATLAB Function/2(Bat_Rate)
  Demux/2 -> MATLAB Function/3(Cap_Rate)
  [Cap_SOC] -> MATLAB Function/4(Cap_SOC)
  [Bat_SOC] -> MATLAB Function/5(Bat_SOC)
  MATLAB Function/1(B_Rate) -> [B_Rate], Product/1
  MATLAB Function/2(C_Rate) -> [C_Rate], Product1/1
  MATLAB Function/3(Cap_over_discharge) -> [Cap_over_discharge]
  MATLAB Function/4(Bat_over_discharge) -> [Bat_over_discharge]
  MATLAB Function/5(Cap_over_charge) -> [Cap_over_charge]
  MATLAB Function/6(Bat_over_charge) -> [Bat_over_charge]
  Saturation3/1 -> [Cap_Charge_Avg]
  MATLAB Function5/3(r2) -> [r3]
  MATLAB Function5/4(r3) -> [r4]
  MATLAB Function5/6(Total_Reward) -> Unit Delay1/1
  [r1] -> Scope1/1  "mid reward"
  [r2] -> Scope1/2  "r1"
  [r3] -> Scope1/3  "r2"
  [r4] -> Scope1/4  "r3"
  [Reward] -> Scope1/6  "Total"
  Unit Delay1/1 -> [Reward]
  [C_Rate] -> Bus Creator4/1  "C Rate"
  [B_Rate] -> Bus Creator4/2  "B Rate"
  Bus Creator4/1 -> Pwr Split/2
  [Observation] -> Agent/1
  [Reward] -> Agent/2
  [isDone] -> Agent/3
  [Action] -> [RL_Cap_Rate], Bus Creator6/2, Minus/2
  Minus/1 -> [RL_Bat_Rate], Bus Creator6/1
  Constant1/1 -> MATLAB Function1/5(sim_case)
  Clock/1 -> MATLAB Function1/6(current_time)
  Constant2/1 -> Divide/2
  [B_Rate] -> MATLAB Function5/5(B_Rate)  "B Rate"
  [C_Rate] -> MATLAB Function5/6(C_Rate)  "C Rate"
  [Bat_SOC] -> Bus Creator/3
  [Power_Demand] -> Divide/1
  [Pwr_Dmd_Norm] -> Scope4/1, Bus Creator/1
  [Bat_SOC] -> MATLAB Function5/1(Bat_SOC)
  Moving Average1/1 -> Derivative/1, Bus Creator1/1
  Bus Creator1/1 -> Scope/1
  Saturation1/1 -> Moving Average1/1
  Divide/1 -> [Pwr_Dmd_Norm]
  MATLAB Function5/5(r4) -> [r5]
  [r5] -> Scope1/5  "r4"
  Derivative/1 -> [Pwr_Derivative]
  [Pwr_Derivative] -> MATLAB Function5/4(Pwr_Dmd_Derivative)

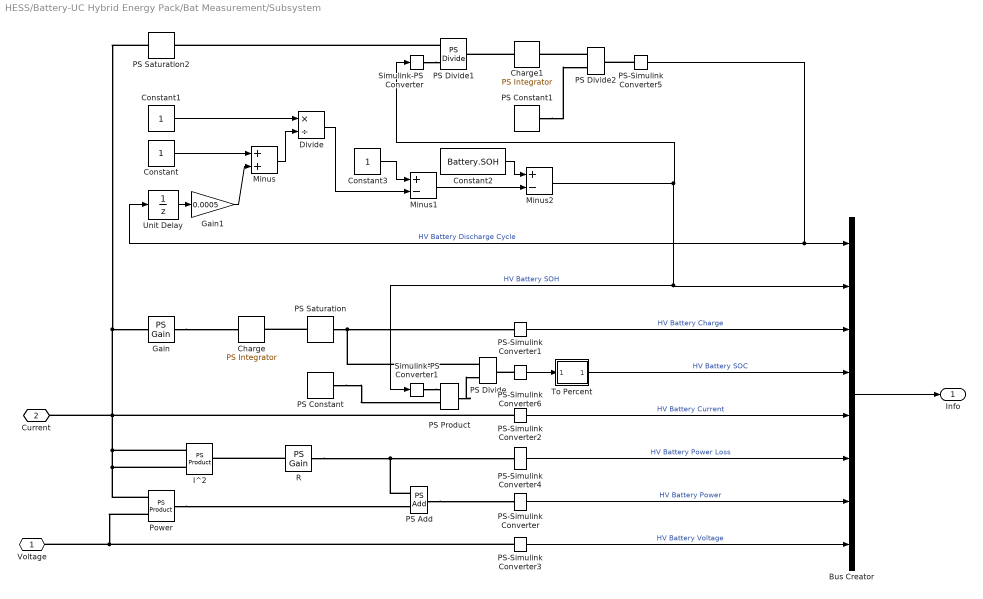
== system HESS/Battery-UC Hybrid Energy Pack/Bat Measurement/Subsystem ==
  Bus Creator : BusCreator  Inputs=8
  Charge : fl_lib/Physical Signals/Linear Operators/PS Integrator  reset_method=foundation.enum.IntegratorResetSpec.None  initial_condition_spec=foundation.enum.IntegratorICSpec.Internal  saturation_spec=foundation.enum.IntegratorSaturationSpec.None  saturation_source_spec=foundation.enum.IntegratorSaturationSourceSpec.Internal  x0=Battery.InitialCharge A*hr  xu=inf s  xl=-inf s
      settings: AttributesFormatString=%<x0> [%<x0_unit>]
  Charge1 : fl_lib/Physical Signals/Linear Operators/PS Integrator  reset_method=foundation.enum.IntegratorResetSpec.None  initial_condition_spec=foundation.enum.IntegratorICSpec.Internal  saturation_spec=foundation.enum.IntegratorSaturationSpec.None  saturation_source_spec=foundation.enum.IntegratorSaturationSourceSpec.Internal  x0=0 A*hr  xu=inf s  xl=-inf s
      settings: AttributesFormatString=%<x0> [%<x0_unit>]
  Constant : Constant
  Constant1 : Constant
  Constant2 : Constant  Value=Battery.SOH
  Constant3 : Constant
  Divide : Product  Inputs=*/
  Gain : fl_lib/Physical Signals/Functions/PS Gain  gain=-1
      settings: AttributesFormatString=%<gain>
  Gain1 : Gain  Gain=0.0005
  I^2 : fl_lib/Physical Signals/Functions/PS Product
  Minus : Sum
  Minus1 : Sum  Inputs=+-
  Minus2 : Sum  Inputs=+-
  PS Add : fl_lib/Physical Signals/Functions/PS Add
  PS Constant : fl_lib/Physical Signals/Sources/PS Constant  constant=Battery.Capacity A*hr
      settings: AttributesFormatString=%<constant> [%<constant_unit>]
  PS Constant1 : fl_lib/Physical Signals/Sources/PS Constant  constant=Battery.Capacity A*hr
  PS Divide : fl_lib/Physical Signals/Functions/PS Divide
  PS Divide1 : fl_lib/Physical Signals/Functions/PS Divide
  PS Divide2 : fl_lib/Physical Signals/Functions/PS Divide
  PS Product : fl_lib/Physical Signals/Functions/PS Product
  PS Saturation : fl_lib/Physical Signals/Nonlinear Operators/PS Saturation  upper_limit=Battery.Capacity A*hr  lower_limit=0 A*hr
      settings: AttributesFormatString=|
      | Upper: %<upper_limit>
      | Lower: %<lower_limit>
  PS Saturation2 : fl_lib/Physical Signals/Nonlinear Operators/PS Saturation  upper_limit=500 A  lower_limit=0 A
  PS-Simulink Converter : nesl_utility/PS-Simulink Converter  PhysicalDomain=network_engine_domain  SubClassName=ps_output  LeftPortType=input  RightPortType=output  PseudoPeriodic=off  Frequencies=[]  VectorFormat=1-D array  Unit=W  AffineConversion=off
  PS-Simulink Converter1 : nesl_utility/PS-Simulink Converter  PhysicalDomain=network_engine_domain  SubClassName=ps_output  LeftPortType=input  RightPortType=output  PseudoPeriodic=off  Frequencies=[]  VectorFormat=1-D array  Unit=A*hr  AffineConversion=off
  PS-Simulink Converter2 : nesl_utility/PS-Simulink Converter  PhysicalDomain=network_engine_domain  SubClassName=ps_output  LeftPortType=input  RightPortType=output  PseudoPeriodic=off  Frequencies=[]  VectorFormat=1-D array  Unit=A  AffineConversion=off
  PS-Simulink Converter3 : nesl_utility/PS-Simulink Converter  PhysicalDomain=network_engine_domain  SubClassName=ps_output  LeftPortType=input  RightPortType=output  PseudoPeriodic=off  Frequencies=[]  VectorFormat=1-D array  Unit=V  AffineConversion=off
  PS-Simulink Converter4 : nesl_utility/PS-Simulink Converter  PhysicalDomain=network_engine_domain  SubClassName=ps_output  LeftPortType=input  RightPortType=output  PseudoPeriodic=off  Frequencies=[]  VectorFormat=1-D array  Unit=W  AffineConversion=off
  PS-Simulink Converter5 : nesl_utility/PS-Simulink Converter  PhysicalDomain=network_engine_domain  SubClassName=ps_output  LeftPortType=input  RightPortType=output  PseudoPeriodic=off  Frequencies=[]  VectorFormat=inherit  Unit=1  AffineConversion=off
  PS-Simulink Converter6 : nesl_utility/PS-Simulink Converter  PhysicalDomain=network_engine_domain  SubClassName=ps_output  LeftPortType=input  RightPortType=output  PseudoPeriodic=off  Frequencies=[]  VectorFormat=1-D array  Unit=1  AffineConversion=off
  Power : fl_lib/Physical Signals/Functions/PS Product
  R : fl_lib/Physical Signals/Functions/PS Gain  gain=Battery.InternalResistance Ohm
      settings: AttributesFormatString=%<gain> [%<gain_unit>]
  Simulink-PS Converter : nesl_utility/Simulink-PS Converter  PhysicalDomain=network_engine_domain  SubClassName=ps_input  LeftPortType=input  RightPortType=output  PseudoPeriodic=off  Frequencies=[]  NoiseDistribution=none  NoiseParameters=[]  Unit=1  AffineConversion=off  FilteringAndDerivatives=provide  SimscapeFilterOrder=1  InputFilterTimeConstant=0.001  UdotUserProvided=0
  Simulink-PS Converter1 : nesl_utility/Simulink-PS Converter  PhysicalDomain=network_engine_domain  SubClassName=ps_input  LeftPortType=input  RightPortType=output  PseudoPeriodic=off  Frequencies=[]  NoiseDistribution=none  NoiseParameters=[]  Unit=1  AffineConversion=off  FilteringAndDerivatives=provide  SimscapeFilterOrder=1  InputFilterTimeConstant=0.001  UdotUserProvided=0
  To Percent : Subsystem
  Unit Delay : UnitDelay  SampleTime=-1  HasFrameUpgradeWarning=on
  Voltage : PMIOPort  Side=Left
  Current : PMIOPort  Port=2  Side=Left
  Info : Outport
  wires:
  PS-Simulink Converter4/1 -> Bus Creator/6  "HV Battery Power Loss"
  PS-Simulink Converter3/1 -> Bus Creator/8  "HV Battery Voltage"
  PS-Simulink Converter1/1 -> Bus Creator/3  "HV Battery Charge"
  Bus Creator/1 -> Info/1
  To Percent/1(Out1) -> Bus Creator/4  "HV Battery SOC"
  PS-Simulink Converter/1 -> Bus Creator/7  "HV Battery Power"
  PS-Simulink Converter6/1 -> To Percent/1(In1)
  PS-Simulink Converter2/1 -> Bus Creator/5  "HV Battery Current"
  Constant/1 -> Minus/1
  Gain1/1 -> Minus/2
  Unit Delay/1 -> Gain1/1
  Divide/1 -> Minus1/2
  Constant1/1 -> Divide/1
  Minus/1 -> Divide/2
  PS-Simulink Converter5/1 -> Bus Creator/1, Unit Delay/1  "HV Battery Discharge Cycle"
  Constant3/1 -> Minus1/1
  Constant2/1 -> Minus2/1
  Minus1/1 -> Minus2/2
  Minus2/1 -> Simulink-PS Converter1/1, Bus Creator/2, Simulink-PS Converter/1  "HV Battery SOH"
  connections:
  PS Divide/LConn1 -- PS-Simulink Converter1/LConn1 -- PS Saturation/RConn1
  Power/LConn1 -- Voltage/RConn1 -- PS-Simulink Converter3/LConn1
  R/RConn1 -- PS Add/LConn1 -- PS-Simulink Converter4/LConn1
  Power/LConn2 -- I^2/LConn1 -- Current/RConn1 -- PS Saturation2/LConn1 -- Gain/LConn1 -- PS-Simulink Converter2/LConn1 -- I^2/LConn2
  PS Add/RConn1 -- PS-Simulink Converter/LConn1
  R/LConn1 -- I^2/RConn1
  PS Saturation/LConn1 -- Charge/RConn1
  Gain/RConn1 -- Charge/LConn1
  PS-Simulink Converter6/LConn1 -- PS Divide/RConn1
  Power/RConn1 -- PS Add/LConn2
  PS Divide1/LConn1 -- PS Saturation2/RConn1
  Charge1/LConn1 -- PS Divide1/RConn1
  PS Divide2/LConn1 -- Charge1/RConn1
  PS Constant1/RConn1 -- PS Divide2/LConn2
  PS-Simulink Converter5/LConn1 -- PS Divide2/RConn1
  Simulink-PS Converter/RConn1 -- PS Divide1/LConn2
  PS Product/RConn1 -- PS Divide/LConn2
  PS Constant/RConn1 -- PS Product/LConn2
  Simulink-PS Converter1/RConn1 -- PS Product/LConn1

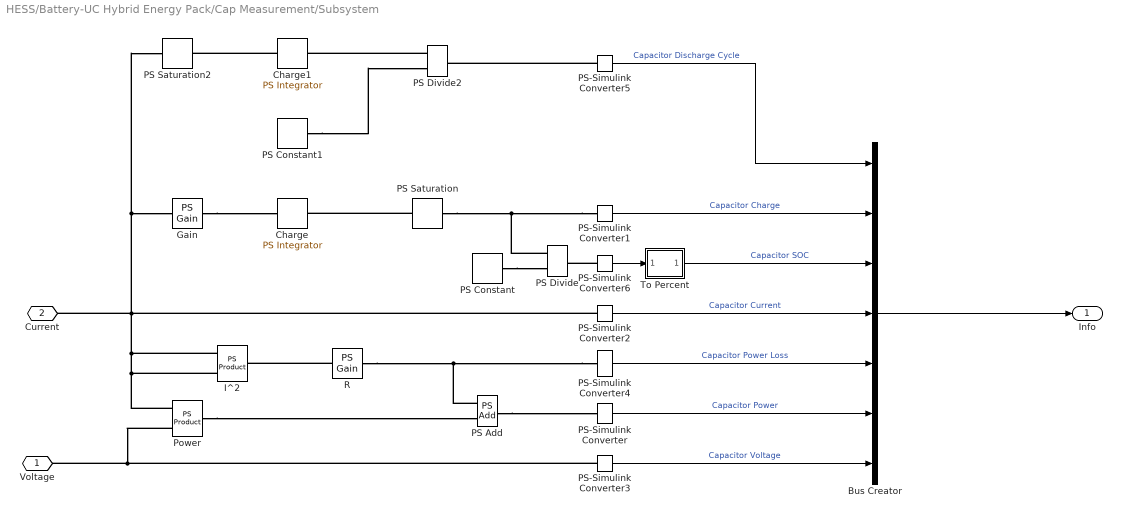
== system HESS/Battery-UC Hybrid Energy Pack/Cap Measurement/Subsystem ==
  Bus Creator : BusCreator  Inputs=7
  Charge : fl_lib/Physical Signals/Linear Operators/PS Integrator  reset_method=foundation.enum.IntegratorResetSpec.None  initial_condition_spec=foundation.enum.IntegratorICSpec.Internal  saturation_spec=foundation.enum.IntegratorSaturationSpec.None  saturation_source_spec=foundation.enum.IntegratorSaturationSourceSpec.Internal  x0=Capacitor.Capacity A*hr  xu=inf s  xl=-inf s
      settings: AttributesFormatString=%<x0> [%<x0_unit>]
  Charge1 : fl_lib/Physical Signals/Linear Operators/PS Integrator  reset_method=foundation.enum.IntegratorResetSpec.None  initial_condition_spec=foundation.enum.IntegratorICSpec.Internal  saturation_spec=foundation.enum.IntegratorSaturationSpec.None  saturation_source_spec=foundation.enum.IntegratorSaturationSourceSpec.Internal  x0=0 A*hr  xu=inf s  xl=-inf s
      settings: AttributesFormatString=%<x0> [%<x0_unit>]
  Gain : fl_lib/Physical Signals/Functions/PS Gain  gain=-1
      settings: AttributesFormatString=%<gain>
  I^2 : fl_lib/Physical Signals/Functions/PS Product
  PS Add : fl_lib/Physical Signals/Functions/PS Add
  PS Constant : fl_lib/Physical Signals/Sources/PS Constant  constant=Capacitor.Capacity A*hr
      settings: AttributesFormatString=%<constant> [%<constant_unit>]
  PS Constant1 : fl_lib/Physical Signals/Sources/PS Constant  constant=Capacitor.Capacity A*hr
      settings: AttributesFormatString=%<constant> [%<constant_unit>]
  PS Divide : fl_lib/Physical Signals/Functions/PS Divide
  PS Divide2 : fl_lib/Physical Signals/Functions/PS Divide
  PS Saturation : fl_lib/Physical Signals/Nonlinear Operators/PS Saturation  upper_limit=Capacitor.Capacity A*hr  lower_limit=0 A*hr
      settings: AttributesFormatString=|
      | Upper: %<upper_limit>
      | Lower: %<lower_limit>
  PS Saturation2 : fl_lib/Physical Signals/Nonlinear Operators/PS Saturation  upper_limit=500 A  lower_limit=0 A
  PS-Simulink Converter : nesl_utility/PS-Simulink Converter  PhysicalDomain=network_engine_domain  SubClassName=ps_output  LeftPortType=input  RightPortType=output  PseudoPeriodic=off  Frequencies=[]  VectorFormat=1-D array  Unit=W  AffineConversion=off
  PS-Simulink Converter1 : nesl_utility/PS-Simulink Converter  PhysicalDomain=network_engine_domain  SubClassName=ps_output  LeftPortType=input  RightPortType=output  PseudoPeriodic=off  Frequencies=[]  VectorFormat=1-D array  Unit=A*hr  AffineConversion=off
  PS-Simulink Converter2 : nesl_utility/PS-Simulink Converter  PhysicalDomain=network_engine_domain  SubClassName=ps_output  LeftPortType=input  RightPortType=output  PseudoPeriodic=off  Frequencies=[]  VectorFormat=1-D array  Unit=A  AffineConversion=off
  PS-Simulink Converter3 : nesl_utility/PS-Simulink Converter  PhysicalDomain=network_engine_domain  SubClassName=ps_output  LeftPortType=input  RightPortType=output  PseudoPeriodic=off  Frequencies=[]  VectorFormat=1-D array  Unit=V  AffineConversion=off
  PS-Simulink Converter4 : nesl_utility/PS-Simulink Converter  PhysicalDomain=network_engine_domain  SubClassName=ps_output  LeftPortType=input  RightPortType=output  PseudoPeriodic=off  Frequencies=[]  VectorFormat=1-D array  Unit=W  AffineConversion=off
  PS-Simulink Converter5 : nesl_utility/PS-Simulink Converter  PhysicalDomain=network_engine_domain  SubClassName=ps_output  LeftPortType=input  RightPortType=output  PseudoPeriodic=off  Frequencies=[]  VectorFormat=inherit  Unit=1  AffineConversion=off
  PS-Simulink Converter6 : nesl_utility/PS-Simulink Converter  PhysicalDomain=network_engine_domain  SubClassName=ps_output  LeftPortType=input  RightPortType=output  PseudoPeriodic=off  Frequencies=[]  VectorFormat=1-D array  Unit=1  AffineConversion=off
  Power : fl_lib/Physical Signals/Functions/PS Product
  R : fl_lib/Physical Signals/Functions/PS Gain  gain=Capacitor.InternalResistance Ohm
      settings: AttributesFormatString=%<gain> [%<gain_unit>]
  To Percent : Subsystem
  Voltage : PMIOPort  Side=Left
  Current : PMIOPort  Port=2  Side=Left
  Info : Outport
  wires:
  PS-Simulink Converter4/1 -> Bus Creator/5  "Capacitor Power Loss"
  PS-Simulink Converter3/1 -> Bus Creator/7  "Capacitor Voltage"
  PS-Simulink Converter1/1 -> Bus Creator/2  "Capacitor Charge"
  Bus Creator/1 -> Info/1
  To Percent/1(Out1) -> Bus Creator/3  "Capacitor SOC"
  PS-Simulink Converter/1 -> Bus Creator/6  "Capacitor Power"
  PS-Simulink Converter6/1 -> To Percent/1(In1)
  PS-Simulink Converter2/1 -> Bus Creator/4  "Capacitor Current"
  PS-Simulink Converter5/1 -> Bus Creator/1  "Capacitor Discharge Cycle"
  connections:
  PS-Simulink Converter1/LConn1 -- PS Divide/LConn1 -- PS Saturation/RConn1
  PS-Simulink Converter3/LConn1 -- Power/LConn1 -- Voltage/RConn1
  PS-Simulink Converter4/LConn1 -- R/RConn1 -- PS Add/LConn1
  Current/RConn1 -- PS Saturation2/LConn1 -- Gain/LConn1 -- PS-Simulink Converter2/LConn1 -- I^2/LConn2 -- I^2/LConn1 -- Power/LConn2
  PS Add/RConn1 -- PS-Simulink Converter/LConn1
  R/LConn1 -- I^2/RConn1
  PS Saturation/LConn1 -- Charge/RConn1
  Gain/RConn1 -- Charge/LConn1
  PS-Simulink Converter6/LConn1 -- PS Divide/RConn1
  Power/RConn1 -- PS Add/LConn2
  PS Constant/RConn1 -- PS Divide/LConn2
  Charge1/LConn1 -- PS Saturation2/RConn1
  PS-Simulink Converter5/LConn1 -- PS Divide2/RConn1
  PS Divide2/LConn1 -- Charge1/RConn1
  PS Constant1/RConn1 -- PS Divide2/LConn2

== system HESS/Battery-UC Hybrid Energy Pack/Bat Measurement/Subsystem/To Percent ==
  In1 : Inport
  Unit Conversion : UnitConversion
  Out1 : Outport  Unit=%
      settings: AttributesFormatString=%<Unit>
  wires:
  Unit Conversion/1 -> Out1/1
  In1/1 -> Unit Conversion/1

== system HESS/Battery-UC Hybrid Energy Pack/Cap Measurement/Subsystem/To Percent ==
  In1 : Inport
  Unit Conversion : UnitConversion
  Out1 : Outport  Unit=%
      settings: AttributesFormatString=%<Unit>
  wires:
  Unit Conversion/1 -> Out1/1
  In1/1 -> Unit Conversion/1

== matlab function HESS/RL-based EMS/SAC/MATLAB Function1 ==
  data: isDone output; Bat_Pwr input; Cap_Pwr input; Pwr_Dmd input; Cap_SOC input; sim_case input; current_time input
function isDone = check(Bat_Pwr, Cap_Pwr, Pwr_Dmd, Cap_SOC, sim_case, current_time)


flag = 0;


if Cap_SOC < 0.2
    flag = 1;
end


if sim_case == 2
    if current_time > 1372
        flag = 1;
    end

elseif sim_case == 3
    if current_time > 1369
        flag = 1;
    end

elseif sim_case == 4
    if current_time > 1022
        flag = 1;
    end

elseif sim_case == 5
    if current_time > 1477
        flag = 1;
    end

elseif sim_case == 6
    if current_time > 1800
        flag = 1;
    end
end

isDone = flag;

== matlab function HESS/RL-based EMS/SAC/MATLAB Function5 ==
  data: Bat_SOC input; reward output; Cap_SOC input; Pwr_Dmd input; Pwr_Dmd_Derivative input; r1 output; r2 output; r3 output; r4 output; Total_Reward output; B_Rate input; C_Rate input
function [reward, r1, r2, r3, r4, Total_Reward] = cal_reward(Bat_SOC, Cap_SOC, Pwr_Dmd, Pwr_Dmd_Derivative, B_Rate, C_Rate)

r1 = 0;
r2 = 0;
r3 = 0;
r4 = 0;

w = Pwr_Dmd / 100000;

reward = Cap_SOC;

% Discharge Reward
if (Cap_SOC > 0.65 && Pwr_Dmd > 0) && (Pwr_Dmd_Derivative > 0)
    r1 = w * C_Rate;
end

% Charge Reward
if (Cap_SOC < 1 && Pwr_Dmd < 0)
    r2 = C_Rate;
end

% Overdischarge Penalty
if Cap_SOC < 0.65 && Pwr_Dmd > 0
    r3 = -2 * (C_Rate);
end

% Overcharge Penalty
if Cap_SOC >= 1 && Pwr_Dmd < 0
    r4 = -2 * (C_Rate);
end

Total_Reward = reward + r1 + r2 + r3 + r4;

== matlab function HESS/RL-based EMS/DQN/MATLAB Function ==
  data: Pwr_Dmd input; Bat_Rate input; B_Rate output; Cap_Rate input; Cap_SOC input; C_Rate output; Cap_over_discharge output; Bat_over_discharge output; Cap_over_charge output; Bat_over_charge output; Bat_SOC input
function [B_Rate, C_Rate, Cap_over_discharge, Bat_over_discharge, Cap_over_charge, Bat_over_charge] = filter(Pwr_Dmd, Bat_Rate, Cap_Rate, Cap_SOC, Bat_SOC)

B_Rate = Bat_Rate;
C_Rate = Cap_Rate;

Bat_over_discharge = 0;
Bat_over_charge = 0;

Cap_over_discharge = 0;
Cap_over_charge = 0;

%{
if (Pwr_Dmd >= 0 && Cap_SOC <= 0.5)

    C_Rate = 0;
    Cap_over_discharge = Cap_Rate;

end

if (Pwr_Dmd >= 0 && Bat_SOC <= 0.2)

    B_Rate = 0;
    Bat_over_discharge = Bat_Rate;

end

if (Pwr_Dmd < 0 && Bat_SOC >= 1)

    B_Rate = 0;
    Bat_over_charge = Bat_Rate;

end

if (Pwr_Dmd < 0 && Cap_SOC >= 1)

    C_Rate = 0;
    Cap_over_charge = Cap_Rate;

end
%}

== matlab function HESS/RL-based EMS/DQN/MATLAB Function1 ==
  data: isDone output; Bat_Pwr input; Cap_Pwr input; Pwr_Dmd input; Cap_SOC input; sim_case input; current_time input
function isDone = check(Bat_Pwr, Cap_Pwr, Pwr_Dmd, Cap_SOC, sim_case, current_time)


flag = 0;


if Cap_SOC < 0.2
    flag = 1;
end


if sim_case == 2
    if current_time > 1372
        flag = 1;
    end

elseif sim_case == 3
    if current_time > 1369
        flag = 1;
    end

elseif sim_case == 4
    if current_time > 1022
        flag = 1;
    end

elseif sim_case == 5
    if current_time > 1477
        flag = 1;
    end

elseif sim_case == 6
    if current_time > 1800
        flag = 1;
    end
end

isDone = flag;

== matlab function HESS/RL-based EMS/DQN/MATLAB Function5 ==
  data: Bat_SOC input; reward output; Cap_SOC input; Pwr_Dmd input; Prev_Pwr_Dmd input; r1 output; r2 output; r3 output; r4 output; Total_Reward output; B_Rate input; C_Rate input
function [reward, r1, r2, r3, r4, Total_Reward] = cal_reward(Bat_SOC, Cap_SOC, Pwr_Dmd, Prev_Pwr_Dmd, B_Rate, C_Rate)

r1 = 0;
r2 = 0;
r3 = 0;
r4 = 0;

w = Pwr_Dmd / 100000;

reward = Cap_SOC;

% Discharge Reward
if (Cap_SOC > 0.65 && Pwr_Dmd > 10000) && (Prev_Pwr_Dmd < Pwr_Dmd)
    r1 = w * C_Rate;
end

% Charge Reward
if (Cap_SOC < 1 && Pwr_Dmd < 0)
    r2 = C_Rate;
end

% Overdischarge Penalty
if Cap_SOC < 0.65 && Pwr_Dmd > 0
    r3 = -(C_Rate);
end

% Overcharge Penalty
if Cap_SOC >= 1 && Pwr_Dmd < 0
    r4 = -(C_Rate);
end

Total_Reward = reward + r1 + r2 + r3 + r4;

== matlab function HESS/RL-based EMS/DQN/MATLAB Function2 ==
  data: Action input; bat_rate output; cap_rate output
function [bat_rate, cap_rate]= fcn(Action)

% Action means cap rate (1 ~ 11)
flag = Action - 1; % (0, 1, 2, 3, 4, 5, 6, 7, 8, 9, 10)

cap_rate = flag * 0.1;
bat_rate = 1 - cap_rate;
